simulink model "CM300A_Adc0CfgAndUse"  (R2013b)
settings: Solver=FixedStepDiscrete  SolverMode=SingleTasking  StartTime=0.0  StopTime=1  FixedStep=0.002  RelTol=1e-3
values from neighbouring files (symbols this model uses):
  ADC0CFGANDUSE_DIAGCSCANGROUPMAX_CNT_U08 = DataDict.Constant    [CM300A_ADC0CfgAndUse_DataDict.m]
  ADC0CFGANDUSE_DIAGCSCANGROUPMIN_CNT_U08 = DataDict.Constant    [CM300A_ADC0CfgAndUse_DataDict.m]
undefined symbols (not defined in the file or in its folder): sigbuilder_block
libraries: simulink x1
settings Model: Creator=nz3zln  LastModifiedBy=wzvp6q
settings SolverCC: AutoInsertRateTranBlk=on  InsertRTBMode=Always
settings DataIOCC: LimitDataPoints=off  SaveFormat=Structure  ReturnWorkspaceOutputs=on
settings OptimizationCC: BlockReduction=off  InlineParams=on  ZeroExternalMemoryAtStartup=off  ZeroInternalMemoryAtStartup=off  OptimizeModelRefInitCode=on  LifeSpan=1
settings DebuggingCC: SignalInfNanChecking=error  SignalRangeChecking=warning  UnderspecifiedInitializationDetection=Simplified  SolverPrmCheckMsg=error  MultiTaskCondExecSysMsg=warning  MultiTaskRateTransMsg=warning  SingleTaskRateTransMsg=warning  CheckMatrixSingularityMsg=error  ParameterUnderflowMsg=error  ParameterPrecisionLossMsg=error  ParameterTunabilityLossMsg=error  FixptConstUnderflowMsg=warning  FixptConstOverflowMsg=warning  VectorMatrixConversionMsg=error  SignalLabelMismatchMsg=error  UnconnectedInputMsg=error  UnconnectedOutputMsg=error  UnconnectedLineMsg=error  SFcnCompatibilityMsg=error  UniqueDataStoreMsg=warning  BusObjectLabelMismatch=error  RootOutportRequireBusObject=error  AssertControl=DisableAll  ModelReferenceIOMsg=error  ModelReferenceVersionMismatchMessage=warning  ModelReferenceIOMismatchMessage=error  ModelReferenceCSMismatchMessage=warning  ModelReferenceDataLoggingMessage=error  StateNameClashWarn=warning  StrictBusMsg=ErrorOnBusTreatedAsVector  NonBusSignalsTreatedAsBus=error  SFUnexpectedBacktrackingDiag=error  SFInvalidInputDataAccessInChartInitDiag=error  SFNoUnconditionalDefaultTransitionDiag=error  SFTransitionOutsideNaturalParentDiag=error  SFUnconditionalTransitionShadowingDiag=error  SFUndirectedBroadcastEventsDiag=error
settings ModelReferenceCC: ModelReferenceNumInstancesAllowed=Single
settings RTWCC: SystemTargetFile=autosar.tlc  GenCodeOnly=on  TemplateMakefile=ert_default_tmf  Description=AUTOSAR  GenerateReport=on  ProcessScript=autosar_make_rtw_hook  LaunchReport=on
settings CodeAppCC: GenerateComments=off  IgnoreCustomStorageClasses=off  CustomSymbolStrType=$N$R$M  CustomSymbolStrBlkIO=$N$M  SimulinkBlockComments=off
settings STFCustomTargetCC: ParMdlRefBuildCompliant=on  CompOptLevelCompliant=on  IncludeMdlTerminateFcn=off  CombineOutputUpdateFcns=on  SuppressErrorStatus=on  ERTFirstTimeCompliant=on  ERTCustomFileBanners=on  SupportNonFinite=off  SupportComplex=off  SupportContinuousTime=off  SupportNonInlinedSFcns=off  MATLABClassNameForMDSCustomization=Simulink.SoftwareTarget.ERTCustomization  AutosarCompliant=on  GRTInterface=off  SystemTargetFile=autosar.tlc
settings ERTTargetCC: CodeReplacementLibrary=ANSI_C  ConcurrentExecutionCompliant=off  IncludeMdlTerminateFcn=off  SuppressErrorStatus=on  SupportNonFinite=off  SupportComplex=off  ModelStepFunctionPrototypeControlCompliant=off  CPPClassGenCompliant=off  AutosarCompliant=on  InlinedParameterPlacement=NonHierarchical  ERTCustomFileTemplate=example_file_process.tlc  EnableUserReplacementTypes=on

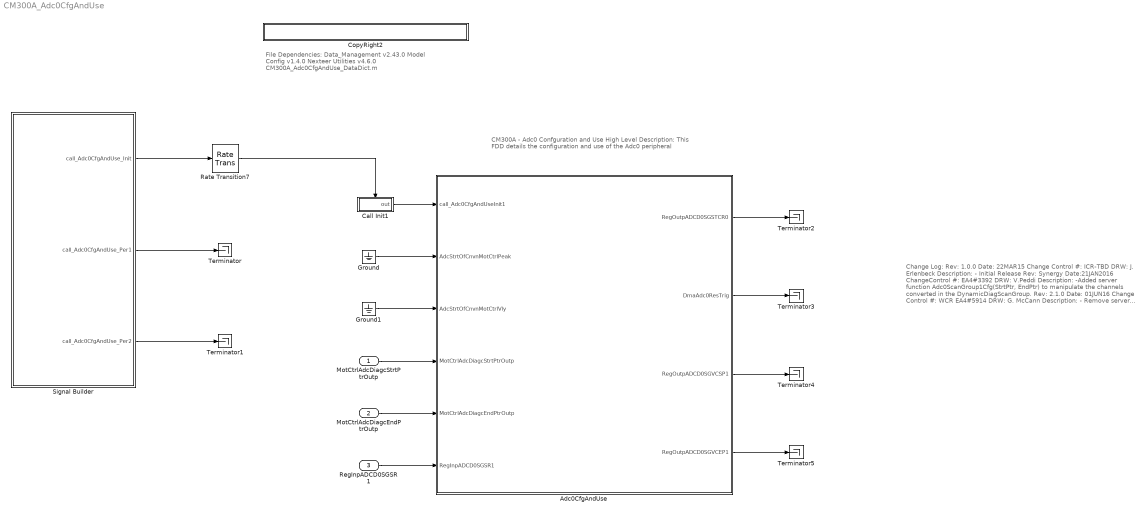
== system CM300A_Adc0CfgAndUse ==
  note: CM300A - Adc0 Confguration and Use
      |
      | High Level Description:
      | This FDD details the configuration and use of the Adc0 peripheral
  note: Change Log:
      |
      | Rev: 1.0.0
      | Date: 22MAR15
      | Change Control #: ICR-TBD
      | DRW: J. Erlenbeck
      | Description:
      | - Initial Release
      |
      | Rev: Synergy
      | Date:21JAN2016
      | ChangeControl #: EA4#3392
      | DRW: V.Peddi
      | Description:
      | -Added server function Adc0ScanGroup1Cfg(StrtPtr, EndPtr)
      |  to manipulate the channels converted in the DynamicDiagScanGroup.
      |
      | Rev: 2.1.0
      | Date: 01JUN16
      | Change Control #: WCR EA4#5914
      | DRW: G. McCann
      | Description:
      | - Remove server function Adc0ScanGroup1Cfg(StrtPtr, EndPtr) and
      |   replace with Adc0CfgAndUsePer1
      | - Make StrtPtr and EndPtr update dependent on a change in inputs and
      |   A/D converter idle state
      |
      | Rev: 2.2.0
      | Date: 07SEP16
      | Change Control #: WCR EA4#7445
      | DRW: G. McCann
      | Description:
      | - Initialize Adc0DiagcStrtPtr and Adc0DiagcEndPtr in Adc0CfgAndUseInit1
      | - Connected I/O to allow model to run without errors
  note: File Dependencies:
      | Data_Management v2.43.0
      | Model Config v1.4.0
      | Nexteer Utilities v4.6.0
      | CM300A_Adc0CfgAndUse_DataDict.m
  MotCtrlAdcDiagcStrtPtrOutp : Inport
  MotCtrlAdcDiagcEndPtrOutp : Inport  Port=2
  RegInpADCD0SGSR1 : Inport  RequirementInfo={} %GIDa_799c9861_6893_4cfe_b57e_ab21633d01ad  Port=3
  Adc0CfgAndUse : Subsystem
  Call Init1 : Subsystem  TreatAsAtomicUnit=on
  CopyRight2 : Subsystem  Description=|  mask(Copyright Information){none=on}
      | Copyright info block.                                               
      |                                                                     
      | Place copyright information at the top of every subsystem in design.
      mask prompts: none "No parameters"
      mask help: Place copyright information at the top of every subsystem in design.
      mask Display:
      | NxtrConf = 'Nexteer Confidential';
      | 
      | sys = bdroot; %handle for the current model ("system")
      | first = get_param(sys,'Created');
      | first = first(end-3:end);  %year is last four digits
      | 
      | last = get_param(sys,'LastModifiedDate');
      | if isempty(last)
      |     last = datestr(now,'yyyy');
      | else
      |     last = last(end-3:end);
      | end
      | 
      | if strcmp(first,last)
      |     fprintf('%s -- Copyright %s Nexteer',NxtrConf,first)
      | else
      |     fprintf('%s -- %s%s- %s Nexteer',NxtrConf,char(169),first,last)
      | end
  Ground : Ground
  Ground1 : Ground
  Rate Transition7 : RateTransition
  Signal Builder : Subsystem  Tag=STV Subsys  RequirementInfo={} %GIDa_2822100e_29fa_4197_9ccc_01864625f252  LoadFcn=sigbuilder_block('load');  StartFcn=sigbuilder_block('start');  StopFcn=sigbuilder_block('stop');  ClipboardFcn=sigbuilder_block('clipboard');  mask(Sigbuilder block){}
      mask help: Simulink:masks:SigbuilderBlock_MD
      mask init:
      | if ~strcmp(get_param(bdroot(gcbh),'SimulationStatus'),'stopped') tuvar = sigbuilder_block('maskInit'); end
      settings: CopyFcn=sigbuilder_block('copy');  DeleteFcn=sigbuilder_block('delete');  ModelCloseFcn=sigbuilder_block('modelClose');  PreSaveFcn=sigbuilder_block('preSave');  PauseFcn=sigbuilder_block('pause');  ContinueFcn=sigbuilder_block('continue');  NameChangeFcn=sigbuilder_block('namechange');  OpenFcn=sigbuilder_block('open',[0 127.5 768 484.5 ]);  CloseFcn=sigbuilder_block('close');
      mask Display: plot(0, 0, 100, 100,[2, 2, 32, 32, 2], [68, 8, 8, 68, 68],[32, 2], [38, 38], [32, 19, 2],[53, 60, 44], [32, 17, 17, 2],[16, 16, 31, 31]);txt = getActiveGroup(gcbh);text(2, 100, txt,'verticalAlignment', 'top');
  Terminator{,1..5} (6 alike) : Terminator
  wires:
  Signal Builder/1(call_Adc0CfgAndUse_Init) -> Rate Transition7/1
  Call Init1/1(out) -> Adc0CfgAndUse/1(call_Adc0CfgAndUseInit1)
  Rate Transition7/1 -> Call Init1/Enable
  Signal Builder/2(call_Adc0CfgAndUse_Per1) -> Terminator/1
  Signal Builder/3(call_Adc0CfgAndUse_Per2) -> Terminator1/1
  MotCtrlAdcDiagcStrtPtrOutp/1 -> Adc0CfgAndUse/4(MotCtrlAdcDiagcStrtPtrOutp)
  MotCtrlAdcDiagcEndPtrOutp/1 -> Adc0CfgAndUse/5(MotCtrlAdcDiagcEndPtrOutp)
  RegInpADCD0SGSR1/1 -> Adc0CfgAndUse/6(RegInpADCD0SGSR1)
  Ground/1 -> Adc0CfgAndUse/2(AdcStrtOfCnvnMotCtrlPeak)
  Ground1/1 -> Adc0CfgAndUse/3(AdcStrtOfCnvnMotCtrlVly)
  Adc0CfgAndUse/1(RegOutpADCD0SGSTCR0) -> Terminator2/1
  Adc0CfgAndUse/2(DmaAdc0ResTrig) -> Terminator3/1
  Adc0CfgAndUse/3(RegOutpADCD0SGVCSP1) -> Terminator4/1
  Adc0CfgAndUse/4(RegOutpADCD0SGVCEP1) -> Terminator5/1

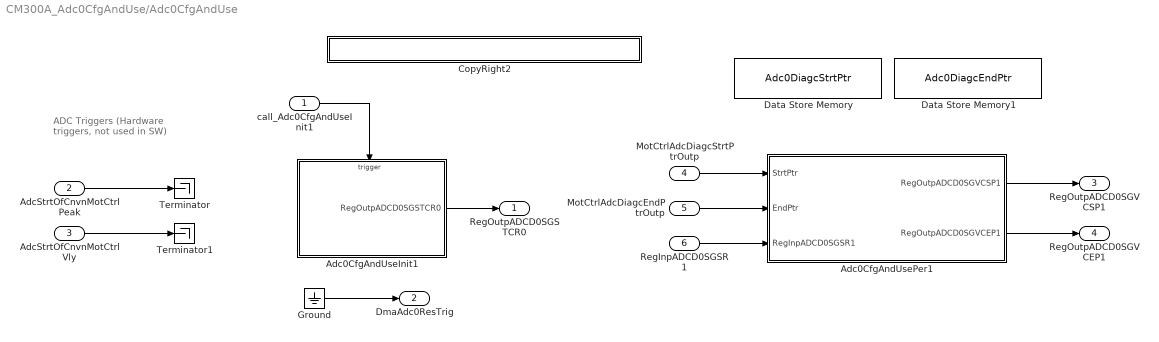
== system CM300A_Adc0CfgAndUse/Adc0CfgAndUse ==
  note: ADC Triggers
      | (Hardware triggers, not used
      | in SW)
  call_Adc0CfgAndUseInit1 : Inport
  AdcStrtOfCnvnMotCtrlPeak : Inport  Port=2
  AdcStrtOfCnvnMotCtrlVly : Inport  Port=3
  MotCtrlAdcDiagcStrtPtrOutp : Inport  RequirementInfo={} %GIDa_ef690fd5_db03_45c7_ba36_4d8aaa37a154  Port=4
  MotCtrlAdcDiagcEndPtrOutp : Inport  RequirementInfo={} %GIDa_8ad929bf_df42_4e40_9b61_eea1733fe1b0  Port=5
  RegInpADCD0SGSR1 : Inport  RequirementInfo={} %GIDa_439b9fca_7ff1_4c84_809f_d1b219b17d54  Port=6
  Adc0CfgAndUseInit1 : Subsystem
  Adc0CfgAndUsePer1 : Subsystem  RequirementInfo="{'linktype_rmi_doors' '0000c472 (/ESG Group/FDD Module Requirements/EA4 Specific/CM300A_Adc0CfgAndUse)' '#CM300A_77' 'true' 'REQ:  CM300A_77' '' } %GIDa_f9ac3182_66c5_4389_b7a8_b1b52d0fa510"
  CopyRight2 : Subsystem  Description=|  mask(Copyright Information){none=on}
      | Copyright info block.                                               
      |                                                                     
      | Place copyright information at the top of every subsystem in design.
      mask prompts: none "No parameters"
      mask help: Place copyright information at the top of every subsystem in design.
      mask Display:
      | NxtrConf = 'Nexteer Confidential';
      | 
      | sys = bdroot; %handle for the current model ("system")
      | first = get_param(sys,'Created');
      | first = first(end-3:end);  %year is last four digits
      | 
      | last = get_param(sys,'LastModifiedDate');
      | if isempty(last)
      |     last = datestr(now,'yyyy');
      | else
      |     last = last(end-3:end);
      | end
      | 
      | if strcmp(first,last)
      |     fprintf('%s -- Copyright %s Nexteer',NxtrConf,first)
      | else
      |     fprintf('%s -- %s%s- %s Nexteer',NxtrConf,char(169),first,last)
      | end
  Data Store Memory : DataStoreMemory  DataStoreName=Adc0DiagcStrtPtr  StateMustResolveToSignalObject=on
  Data Store Memory1 : DataStoreMemory  DataStoreName=Adc0DiagcEndPtr  StateMustResolveToSignalObject=on
  Ground : Ground
  Terminator : Terminator
  Terminator1 : Terminator
  RegOutpADCD0SGSTCR0 : Outport  RequirementInfo={} %GIDa_38330155_36ba_489f_82a9_9da59df6df64
  DmaAdc0ResTrig : Outport  RequirementInfo={'linktype_rmi_doors' '0000c472 (/ESG Group/FDD Module Requirements/EA4 Specific/CM300A_Adc0CfgAndUse)' '#CM300A_84' 'true' 'REQ: CM300A_84' '' } %GIDa_96a67154_1cf8_4536_bab5_cb4a5a0ca20a  Port=2
  RegOutpADCD0SGVCSP1 : Outport  Port=3
  RegOutpADCD0SGVCEP1 : Outport  Port=4
  wires:
  call_Adc0CfgAndUseInit1/1 -> Adc0CfgAndUseInit1/Trigger
  Adc0CfgAndUseInit1/1(RegOutpADCD0SGSTCR0) -> RegOutpADCD0SGSTCR0/1
  AdcStrtOfCnvnMotCtrlPeak/1 -> Terminator/1
  AdcStrtOfCnvnMotCtrlVly/1 -> Terminator1/1
  Ground/1 -> DmaAdc0ResTrig/1
  MotCtrlAdcDiagcStrtPtrOutp/1 -> Adc0CfgAndUsePer1/1(StrtPtr)
  MotCtrlAdcDiagcEndPtrOutp/1 -> Adc0CfgAndUsePer1/2(EndPtr)
  Adc0CfgAndUsePer1/1(RegOutpADCD0SGVCSP1) -> RegOutpADCD0SGVCSP1/1
  Adc0CfgAndUsePer1/2(RegOutpADCD0SGVCEP1) -> RegOutpADCD0SGVCEP1/1
  RegInpADCD0SGSR1/1 -> Adc0CfgAndUsePer1/3(RegInpADCD0SGSR1)

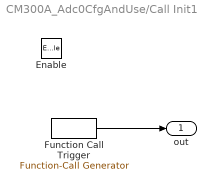
== system CM300A_Adc0CfgAndUse/Call Init1 ==
  Enable : EnablePort
  Function Call Trigger : simulink/Ports & Subsystems/Function-Call Generator  RequirementInfo="{'linktype_rmi_doors' '000089e3 (/E-STEER_New/System Specification Documents/Core Specs/Subsystem Specs/System Functions FDD/SF-46  Gross Cross Check)' '#211' 'true' '3.1-1 The GCC function shall monitor every posted output motor comm' '' ; 'linktype_rmi_doors' '000089e3 (/E-STEER_New/System Specification Documents/Core Specs/Subsystem Specs/System Functions FDD/SF-46  Gross Cross Check)' '#182' 'true' '3.2.2-1 GCC shall be executed at a 0.002 second loop time.' '' } %GIDa_ff755a2e_49d1_45f7_8591_3ce0ef475338"  sample_time=0.002  numberOfIterations=1
  out : Outport
  wires:
  Function Call Trigger/1 -> out/1

== system CM300A_Adc0CfgAndUse/CopyRight2 ==

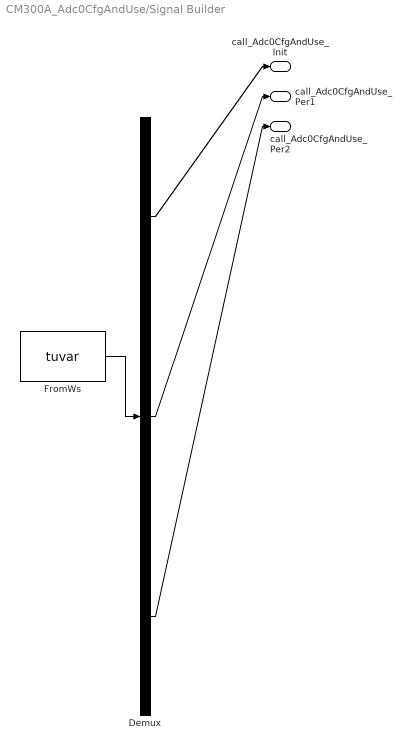
== system CM300A_Adc0CfgAndUse/Signal Builder ==
  Demux : Demux  Tag=STV Demux  Outputs=3
  FromWs : FromWorkspace  Tag=STV FromWs  VariableName=tuvar  SampleTime=0
      SigBuilderData=|
      | common.afterFinalStr = 'Extrapolate'
      | common.sampleTime = 0
      | dataSet(1).timeRange = [0 0.5]
      | dataSet(1).name = 'Group 1'
      | dataSet(2).timeRange = [0 0.5]
      | dataSet(2).name = 'Group 2'
      | dataSet(3).timeRange = [0 1.2]
      | dataSet(3).name = 'Group 3'
      | dataSet(4).timeRange = [0 5]
      | dataSet(4).name = 'Group 4'
      | dataSet(5).timeRange = [0 10]
      | dataSet(5).name = 'Group 5'
      | dataSet(6).timeRange = [0 8]
      | dataSet(6).name = 'Group 6'
      | sbobj.Groups(1).Name = 'Group 1'
      | sbobj.Groups(1).Signals(1).Name = 'call_Adc0CfgAndUse_Init'
      | sbobj.Groups(1).Signals(1).XData = [0 0.001 0.001 0.5]
      | sbobj.Groups(1).Signals(1).YData = [1 1 0 0]
      | sbobj.Groups(1).Signals(2).Name = 'call_Adc0CfgAndUse_Per1'
      | sbobj.Groups(1).Signals(2).XData = [0 0.002 0.002 0.5]
      | sbobj.Groups(1).Signals(2).YData = [0 0 1 1]
      | sbobj.Groups(1).Signals(3).Name = 'call_Adc0CfgAndUse_Per2'
      | sbobj.Groups(1).Signals(3).XData = [0 0.002 0.002 8]
      | sbobj.Groups(1).Signals(3).YData = [0 0 1 1]
      | sbobj.Groups(1).TimeRange = [0 0.5]
      | sbobj.Groups(2).Name = 'Group 2'
      | sbobj.Groups(2).Signals(1).Name = 'call_Adc0CfgAndUse_Init'
      | sbobj.Groups(2).Signals(1).XData = [0 0.001 0.001 0.5]
      | sbobj.Groups(2).Signals(1).YData = [1 1 0 0]
      | sbobj.Groups(2).Signals(2).Name = 'call_Adc0CfgAndUse_Per1'
      | sbobj.Groups(2).Signals(2).XData = [0 0.002 0.002 0.5]
      | sbobj.Groups(2).Signals(2).YData = [0 0 1 1]
      | sbobj.Groups(2).Signals(3).Name = 'call_Adc0CfgAndUse_Per2'
      | sbobj.Groups(2).Signals(3).XData = [0 0.002 0.002 8]
      | sbobj.Groups(2).Signals(3).YData = [0 0 1 1]
      | sbobj.Groups(2).TimeRange = [0 0.5]
      | sbobj.Groups(3).Name = 'Group 3'
      | sbobj.Groups(3).Signals(1).Name = 'call_Adc0CfgAndUse_Init'
      | sbobj.Groups(3).Signals(1).XData = [0 0.001 0.001 1.2]
      | sbobj.Groups(3).Signals(1).YData = [1 1 0 0]
      | sbobj.Groups(3).Signals(2).Name = 'call_Adc0CfgAndUse_Per1'
      | sbobj.Groups(3).Signals(2).XData = [0 0.002 0.002 1.2]
      | sbobj.Groups(3).Signals(2).YData = [0 0 1 1]
      | sbobj.Groups(3).Signals(3).Name = 'call_Adc0CfgAndUse_Per2'
      | sbobj.Groups(3).Signals(3).XData = [0 0.002 0.002 8]
      | sbobj.Groups(3).Signals(3).YData = [0 0 1 1]
      | sbobj.Groups(3).TimeRange = [0 1.2]
      | sbobj.Groups(4).Name = 'Group 4'
      | sbobj.Groups(4).Signals(1).Name = 'call_Adc0CfgAndUse_Init'
      | sbobj.Groups(4).Signals(1).XData = [0 0.001 0.001 5]
      | sbobj.Groups(4).Signals(1).YData = [1 1 0 0]
      | sbobj.Groups(4).Signals(2).Name = 'call_Adc0CfgAndUse_Per1'
      | sbobj.Groups(4).Signals(2).XData = [0 0.002 0.002 5]
      | sbobj.Groups(4).Signals(2).YData = [0 0 1 1]
      | sbobj.Groups(4).Signals(3).Name = 'call_Adc0CfgAndUse_Per2'
      | sbobj.Groups(4).Signals(3).XData = [0 0.002 0.002 8]
      | sbobj.Groups(4).Signals(3).YData = [0 0 1 1]
      | sbobj.Groups(4).TimeRange = [0 5]
      | sbobj.Groups(5).Name = 'Group 5'
      | sbobj.Groups(5).Signals(1).Name = 'call_Adc0CfgAndUse_Init'
      | sbobj.Groups(5).Signals(1).XData = [0 0.001 0.001 10]
      | sbobj.Groups(5).Signals(1).YData = [1 1 0 0]
      | sbobj.Groups(5).Signals(2).Name = 'call_Adc0CfgAndUse_Per1'
      | sbobj.Groups(5).Signals(2).XData = [0 0.002 0.002 10]
      | sbobj.Groups(5).Signals(2).YData = [0 0 1 1]
      | sbobj.Groups(5).Signals(3).Name = 'call_Adc0CfgAndUse_Per2'
      | sbobj.Groups(5).Signals(3).XData = [0 0.002 0.002 10]
      | sbobj.Groups(5).Signals(3).YData = [0 0 1 1]
      | sbobj.Groups(6).Name = 'Group 6'
      | sbobj.Groups(6).Signals(1).Name = 'call_Adc0CfgAndUse_Init'
      | sbobj.Groups(6).Signals(1).XData = [0 0.001 0.001 8]
      | sbobj.Groups(6).Signals(1).YData = [1 1 0 0]
      | sbobj.Groups(6).Signals(2).Name = 'call_Adc0CfgAndUse_Per1'
      | sbobj.Groups(6).Signals(2).XData = [0 0.002 0.002 8]
      | sbobj.Groups(6).Signals(2).YData = [0 0 1 1]
      | sbobj.Groups(6).Signals(3).Name = 'call_Adc0CfgAndUse_Per2'
      | sbobj.Groups(6).Signals(3).XData = [0 0.002 0.002 8]
      | sbobj.Groups(6).Signals(3).YData = [0 0 1 1]
      | sbobj.Groups(6).TimeRange = [0 8]
  call_Adc0CfgAndUse_Init : Outport  Tag=STV Outport
  call_Adc0CfgAndUse_Per1 : Outport  Tag=STV Outport  Port=2
  call_Adc0CfgAndUse_Per2 : Outport  Tag=STV Outport  Port=3
  wires:
  FromWs/1 -> Demux/1
  Demux/1 -> call_Adc0CfgAndUse_Init/1
  Demux/2 -> call_Adc0CfgAndUse_Per1/1
  Demux/3 -> call_Adc0CfgAndUse_Per2/1

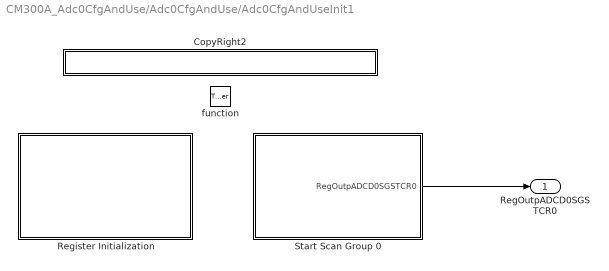
== system CM300A_Adc0CfgAndUse/Adc0CfgAndUse/Adc0CfgAndUseInit1 ==
  function : TriggerPort  TriggerType=function-call
  CopyRight2 : Subsystem  Description=|  mask(Copyright Information){none=on}
      | Copyright info block.                                               
      |                                                                     
      | Place copyright information at the top of every subsystem in design.
      mask prompts: none "No parameters"
      mask help: Place copyright information at the top of every subsystem in design.
      mask Display:
      | NxtrConf = 'Nexteer Confidential';
      | 
      | sys = bdroot; %handle for the current model ("system")
      | first = get_param(sys,'Created');
      | first = first(end-3:end);  %year is last four digits
      | 
      | last = get_param(sys,'LastModifiedDate');
      | if isempty(last)
      |     last = datestr(now,'yyyy');
      | else
      |     last = last(end-3:end);
      | end
      | 
      | if strcmp(first,last)
      |     fprintf('%s -- Copyright %s Nexteer',NxtrConf,first)
      | else
      |     fprintf('%s -- %s%s- %s Nexteer',NxtrConf,char(169),first,last)
      | end
  Register Initialization : Subsystem  Priority=10
      settings: AttributesFormatString=Priority: %<Priority>
  Start Scan Group 0 : Subsystem  RequirementInfo={'linktype_rmi_doors' '0000c472 (/ESG Group/FDD Module Requirements/EA4 Specific/CM300A_Adc0CfgAndUse)' '#CM300A_76' 'true' 'REQ: CM300A_76' '' } %GIDa_d862d82c_969a_40be_9cba_5dad28e4f649  Priority=20
      settings: AttributesFormatString=Priority: %<Priority>
  RegOutpADCD0SGSTCR0 : Outport  RequirementInfo={} %GIDa_29d6058b_2806_49c9_89f2_49c183a99fc2
  wires:
  Start Scan Group 0/1(RegOutpADCD0SGSTCR0) -> RegOutpADCD0SGSTCR0/1

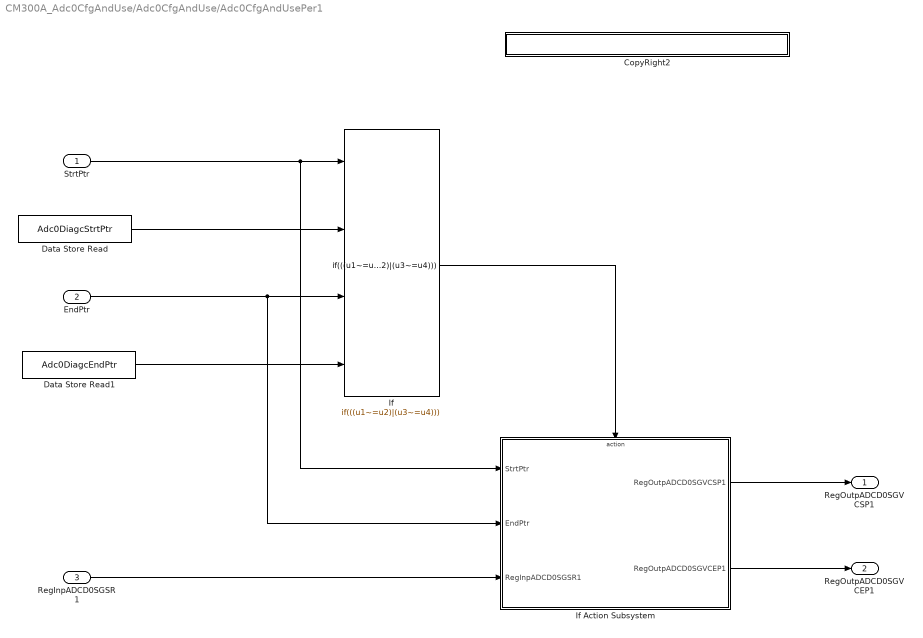
== system CM300A_Adc0CfgAndUse/Adc0CfgAndUse/Adc0CfgAndUsePer1 ==
  StrtPtr : Inport  RequirementInfo="{'linktype_rmi_doors' '0000c472 (/ESG Group/FDD Module Requirements/EA4 Specific/CM300A_Adc0CfgAndUse)' '#CM300A_75' 'true' 'REQ:  CM300A_75' '' } %GIDa_9a820c62_bc96_404d_bb8c_22c729483ef4"
  EndPtr : Inport  RequirementInfo="{'linktype_rmi_doors' '0000c472 (/ESG Group/FDD Module Requirements/EA4 Specific/CM300A_Adc0CfgAndUse)' '#CM300A_75' 'true' 'REQ:  CM300A_75' '' } %GIDa_2d4a3692_8c7d_4d3b_bfda_3dc8696cfa54"  Port=2
  RegInpADCD0SGSR1 : Inport  RequirementInfo={} %GIDa_46fdda9e_6ea4_40cd_8efe_83ccfca36ee1  Port=3
  CopyRight2 : Subsystem  Description=|  mask(Copyright Information){none=on}
      | Copyright info block.                                               
      |                                                                     
      | Place copyright information at the top of every subsystem in design.
      mask prompts: none "No parameters"
      mask help: Place copyright information at the top of every subsystem in design.
      mask Display:
      | NxtrConf = 'Nexteer Confidential';
      | 
      | sys = bdroot; %handle for the current model ("system")
      | first = get_param(sys,'Created');
      | first = first(end-3:end);  %year is last four digits
      | 
      | last = get_param(sys,'LastModifiedDate');
      | if isempty(last)
      |     last = datestr(now,'yyyy');
      | else
      |     last = last(end-3:end);
      | end
      | 
      | if strcmp(first,last)
      |     fprintf('%s -- Copyright %s Nexteer',NxtrConf,first)
      | else
      |     fprintf('%s -- %s%s- %s Nexteer',NxtrConf,char(169),first,last)
      | end
  Data Store Read : DataStoreRead  DataStoreName=Adc0DiagcStrtPtr
  Data Store Read1 : DataStoreRead  DataStoreName=Adc0DiagcEndPtr
  If : If  NumInputs=4  IfExpression=((u1~=u2)|(u3~=u4))  ShowElse=off
  If Action Subsystem : Subsystem  TreatAsAtomicUnit=on
  RegOutpADCD0SGVCSP1 : Outport
  RegOutpADCD0SGVCEP1 : Outport  Port=2
  wires:
  If Action Subsystem/1(RegOutpADCD0SGVCSP1) -> RegOutpADCD0SGVCSP1/1
  If Action Subsystem/2(RegOutpADCD0SGVCEP1) -> RegOutpADCD0SGVCEP1/1
  If/1 -> If Action Subsystem/Action
  StrtPtr/1 -> If Action Subsystem/1(StrtPtr), If/1
  EndPtr/1 -> If Action Subsystem/2(EndPtr), If/3
  RegInpADCD0SGSR1/1 -> If Action Subsystem/3(RegInpADCD0SGSR1)
  Data Store Read/1 -> If/2
  Data Store Read1/1 -> If/4

== system CM300A_Adc0CfgAndUse/Adc0CfgAndUse/CopyRight2 ==

== system CM300A_Adc0CfgAndUse/Adc0CfgAndUse/Adc0CfgAndUseInit1/CopyRight2 ==

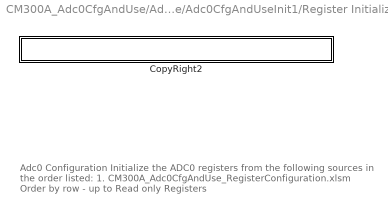
== system CM300A_Adc0CfgAndUse/Adc0CfgAndUse/Adc0CfgAndUseInit1/Register Initialization ==
  note: Adc0 Configuration
      | Initialize the ADC0 registers from the following sources in the order listed:
      |
      | 1. CM300A_Adc0CfgAndUse_RegisterConfiguration.xlsm
      |     Order by row - up to Read only Registers
  CopyRight2 : Subsystem  Description=|  mask(Copyright Information){none=on}
      | Copyright info block.                                               
      |                                                                     
      | Place copyright information at the top of every subsystem in design.
      mask prompts: none "No parameters"
      mask help: Place copyright information at the top of every subsystem in design.
      mask Display:
      | NxtrConf = 'Nexteer Confidential';
      | 
      | sys = bdroot; %handle for the current model ("system")
      | first = get_param(sys,'Created');
      | first = first(end-3:end);  %year is last four digits
      | 
      | last = get_param(sys,'LastModifiedDate');
      | if isempty(last)
      |     last = datestr(now,'yyyy');
      | else
      |     last = last(end-3:end);
      | end
      | 
      | if strcmp(first,last)
      |     fprintf('%s -- Copyright %s Nexteer',NxtrConf,first)
      | else
      |     fprintf('%s -- %s%s- %s Nexteer',NxtrConf,char(169),first,last)
      | end

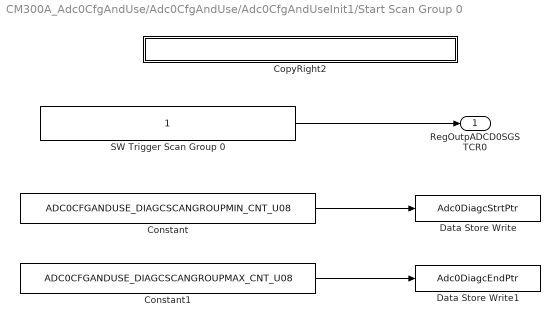
== system CM300A_Adc0CfgAndUse/Adc0CfgAndUse/Adc0CfgAndUseInit1/Start Scan Group 0 ==
  Constant : Constant  Value=ADC0CFGANDUSE_DIAGCSCANGROUPMIN_CNT_U08
  Constant1 : Constant  Value=ADC0CFGANDUSE_DIAGCSCANGROUPMAX_CNT_U08
  CopyRight2 : Subsystem  Description=|  mask(Copyright Information){none=on}
      | Copyright info block.                                               
      |                                                                     
      | Place copyright information at the top of every subsystem in design.
      mask prompts: none "No parameters"
      mask help: Place copyright information at the top of every subsystem in design.
      mask Display:
      | NxtrConf = 'Nexteer Confidential';
      | 
      | sys = bdroot; %handle for the current model ("system")
      | first = get_param(sys,'Created');
      | first = first(end-3:end);  %year is last four digits
      | 
      | last = get_param(sys,'LastModifiedDate');
      | if isempty(last)
      |     last = datestr(now,'yyyy');
      | else
      |     last = last(end-3:end);
      | end
      | 
      | if strcmp(first,last)
      |     fprintf('%s -- Copyright %s Nexteer',NxtrConf,first)
      | else
      |     fprintf('%s -- %s%s- %s Nexteer',NxtrConf,char(169),first,last)
      | end
  Data Store Write : DataStoreWrite  DataStoreName=Adc0DiagcStrtPtr
  Data Store Write1 : DataStoreWrite  DataStoreName=Adc0DiagcEndPtr
  SW Trigger Scan Group 0 : Constant  OutDataTypeStr=uint8
  RegOutpADCD0SGSTCR0 : Outport  RequirementInfo={} %GIDa_c6fe82bc_6768_4bbb_8f71_a05cf9df8531
  wires:
  SW Trigger Scan Group 0/1 -> RegOutpADCD0SGSTCR0/1
  Constant/1 -> Data Store Write/1
  Constant1/1 -> Data Store Write1/1

== system CM300A_Adc0CfgAndUse/Adc0CfgAndUse/Adc0CfgAndUsePer1/CopyRight2 ==

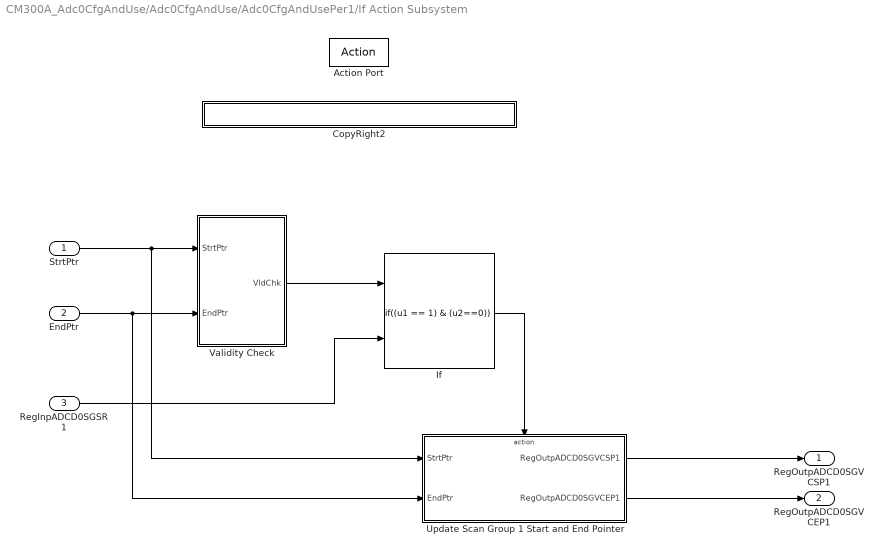
== system CM300A_Adc0CfgAndUse/Adc0CfgAndUse/Adc0CfgAndUsePer1/If Action Subsystem ==
  StrtPtr : Inport  RequirementInfo="{'linktype_rmi_doors' '0000c472 (/ESG Group/FDD Module Requirements/EA4 Specific/CM300A_Adc0CfgAndUse)' '#CM300A_75' 'true' 'REQ:  CM300A_75' '' } %GIDa_022591b1_7db2_42a7_af93_e36ae03ea087"
  EndPtr : Inport  RequirementInfo="{'linktype_rmi_doors' '0000c472 (/ESG Group/FDD Module Requirements/EA4 Specific/CM300A_Adc0CfgAndUse)' '#CM300A_75' 'true' 'REQ:  CM300A_75' '' } %GIDa_b6a3e901_5d29_496c_b383_cce9b5c19cbe"  Port=2
  RegInpADCD0SGSR1 : Inport  RequirementInfo={} %GIDa_280d12e7_dc48_417b_b172_d11a028121ef  Port=3
  Action Port : ActionPort  ActionType=then
  CopyRight2 : Subsystem  Description=|  mask(Copyright Information){none=on}
      | Copyright info block.                                               
      |                                                                     
      | Place copyright information at the top of every subsystem in design.
      mask prompts: none "No parameters"
      mask help: Place copyright information at the top of every subsystem in design.
      mask Display:
      | NxtrConf = 'Nexteer Confidential';
      | 
      | sys = bdroot; %handle for the current model ("system")
      | first = get_param(sys,'Created');
      | first = first(end-3:end);  %year is last four digits
      | 
      | last = get_param(sys,'LastModifiedDate');
      | if isempty(last)
      |     last = datestr(now,'yyyy');
      | else
      |     last = last(end-3:end);
      | end
      | 
      | if strcmp(first,last)
      |     fprintf('%s -- Copyright %s Nexteer',NxtrConf,first)
      | else
      |     fprintf('%s -- %s%s- %s Nexteer',NxtrConf,char(169),first,last)
      | end
  If : If  NumInputs=2  IfExpression=(u1 == 1) & (u2==0)  ShowElse=off
  Update Scan Group 1 Start and End Pointer : Subsystem  RequirementInfo="{'linktype_rmi_doors' '0000c472 (/ESG Group/FDD Module Requirements/EA4 Specific/CM300A_Adc0CfgAndUse)' '#CM300A_94' 'true' 'REQ:  CM300A_94' '' } %GIDa_0212ccd5_1d79_44f0_bbc4_5547b01d16d4"  TreatAsAtomicUnit=on
  Validity Check : Subsystem  RequirementInfo="{'linktype_rmi_doors' '0000c472 (/ESG Group/FDD Module Requirements/EA4 Specific/CM300A_Adc0CfgAndUse)' '#CM300A_75' 'true' 'REQ:  CM300A_75' '' } %GIDa_a2fe9593_817c_42b5_866b_ac4b188cfeca"
  RegOutpADCD0SGVCSP1 : Outport
  RegOutpADCD0SGVCEP1 : Outport  Port=2
  wires:
  If/1 -> Update Scan Group 1 Start and End Pointer/Action
  Update Scan Group 1 Start and End Pointer/1(RegOutpADCD0SGVCSP1) -> RegOutpADCD0SGVCSP1/1
  Update Scan Group 1 Start and End Pointer/2(RegOutpADCD0SGVCEP1) -> RegOutpADCD0SGVCEP1/1
  Validity Check/1(VldChk) -> If/1
  StrtPtr/1 -> Validity Check/1(StrtPtr), Update Scan Group 1 Start and End Pointer/1(StrtPtr)
  EndPtr/1 -> Update Scan Group 1 Start and End Pointer/2(EndPtr), Validity Check/2(EndPtr)
  RegInpADCD0SGSR1/1 -> If/2

== system CM300A_Adc0CfgAndUse/Adc0CfgAndUse/Adc0CfgAndUseInit1/Register Initialization/CopyRight2 ==

== system CM300A_Adc0CfgAndUse/Adc0CfgAndUse/Adc0CfgAndUseInit1/Start Scan Group 0/CopyRight2 ==

== system CM300A_Adc0CfgAndUse/Adc0CfgAndUse/Adc0CfgAndUsePer1/If Action Subsystem/CopyRight2 ==

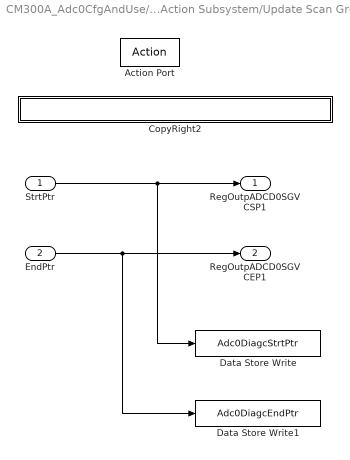
== system CM300A_Adc0CfgAndUse/Adc0CfgAndUse/Adc0CfgAndUsePer1/If Action Subsystem/Update Scan Group 1 Start and End Pointer ==
  StrtPtr : Inport
  EndPtr : Inport  Port=2
  Action Port : ActionPort  ActionType=then
  CopyRight2 : Subsystem  Description=|  mask(Copyright Information){none=on}
      | Copyright info block.                                               
      |                                                                     
      | Place copyright information at the top of every subsystem in design.
      mask prompts: none "No parameters"
      mask help: Place copyright information at the top of every subsystem in design.
      mask Display:
      | NxtrConf = 'Nexteer Confidential';
      | 
      | sys = bdroot; %handle for the current model ("system")
      | first = get_param(sys,'Created');
      | first = first(end-3:end);  %year is last four digits
      | 
      | last = get_param(sys,'LastModifiedDate');
      | if isempty(last)
      |     last = datestr(now,'yyyy');
      | else
      |     last = last(end-3:end);
      | end
      | 
      | if strcmp(first,last)
      |     fprintf('%s -- Copyright %s Nexteer',NxtrConf,first)
      | else
      |     fprintf('%s -- %s%s- %s Nexteer',NxtrConf,char(169),first,last)
      | end
  Data Store Write : DataStoreWrite  DataStoreName=Adc0DiagcStrtPtr
  Data Store Write1 : DataStoreWrite  DataStoreName=Adc0DiagcEndPtr
  RegOutpADCD0SGVCSP1 : Outport
  RegOutpADCD0SGVCEP1 : Outport  Port=2
  wires:
  StrtPtr/1 -> Data Store Write/1, RegOutpADCD0SGVCSP1/1
  EndPtr/1 -> Data Store Write1/1, RegOutpADCD0SGVCEP1/1

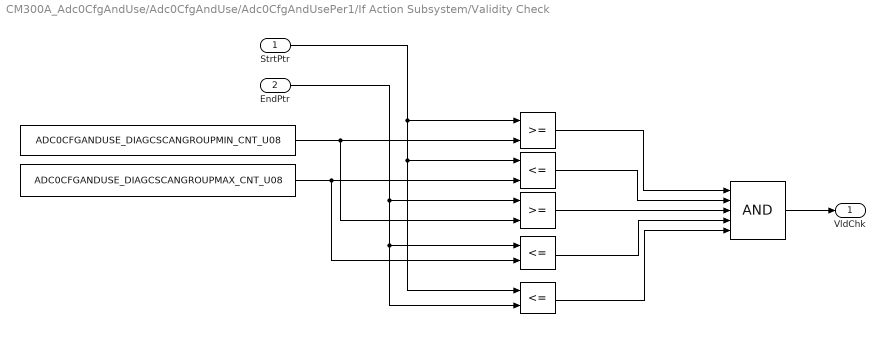
== system CM300A_Adc0CfgAndUse/Adc0CfgAndUse/Adc0CfgAndUsePer1/If Action Subsystem/Validity Check ==
  StrtPtr : Inport  RequirementInfo={} %GIDa_cea07ab8_e198_41bb_96ee_5654fde74799
  EndPtr : Inport  RequirementInfo={} %GIDa_a92a5b44_3f27_4686_bd51_77a48983e70b  Port=2
  " " : Constant  RequirementInfo={} %GIDa_cfa7bfd0_60e7_4ac3_82be_12a7b9be73f4  Value=ADC0CFGANDUSE_DIAGCSCANGROUPMIN_CNT_U08
  "  " : RelationalOperator  RequirementInfo={} %GIDa_bb1ef53a_160a_4e1b_85c6_d3c6ce50273f  OutDataTypeStr=boolean
  "   " : Constant  RequirementInfo={} %GIDa_6b3f91af_3f86_4239_826a_db4197e8aa2b  Value=ADC0CFGANDUSE_DIAGCSCANGROUPMAX_CNT_U08
  "     " : RelationalOperator  RequirementInfo={} %GIDa_96a38213_d20d_40a0_a619_a1de297a20dd  Operator=<=  OutDataTypeStr=boolean
  "      " : RelationalOperator  RequirementInfo={} %GIDa_cf919f57_02da_4f8c_84ae_7ddbabdc6d16  Operator=<=  OutDataTypeStr=boolean
  "       " : RelationalOperator  RequirementInfo={} %GIDa_23d1fcbd_1b75_48ee_9273_825ce088b766  OutDataTypeStr=boolean
  "         " : RelationalOperator  RequirementInfo={} %GIDa_511801bc_adc3_4e34_987f_5557efca4e77  Operator=<=  OutDataTypeStr=boolean
  "          " : Logic  RequirementInfo={} %GIDa_5714c7c3_6138_43b6_9fef_7b29415762af  Inputs=5  AllPortsSameDT=off  OutDataTypeStr=boolean
  VldChk : Outport
  wires:
  "     "/1 -> "          "/4
  " "/1 -> "       "/2, "  "/2
  EndPtr/1 -> "      "/2, "     "/1, "       "/1
  "   "/1 -> "     "/2, "         "/2
  "       "/1 -> "          "/3
  "  "/1 -> "          "/1
  StrtPtr/1 -> "      "/1, "         "/1, "  "/1
  "      "/1 -> "          "/5
  "         "/1 -> "          "/2
  "          "/1 -> VldChk/1

== system CM300A_Adc0CfgAndUse/Adc0CfgAndUse/Adc0CfgAndUsePer1/If Action Subsystem/Update Scan Group 1 Start and End Pointer/CopyRight2 ==
